simulink subsystem "ageing_model"  (R2022a)
settings: Solver=VariableStepAuto  StartTime=0.0  StopTime=10.0  RelTol=1e-3
undefined symbols (not defined in the file): Cn
settings Model: Creator=mateu  LastModifiedBy=mateu

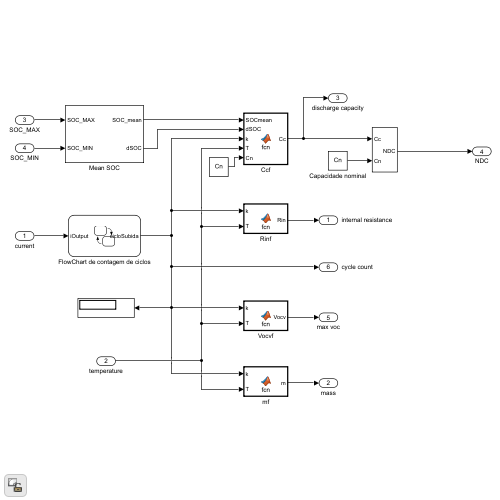
[thumbnail: Simulink's stored preview of the top-level diagram]
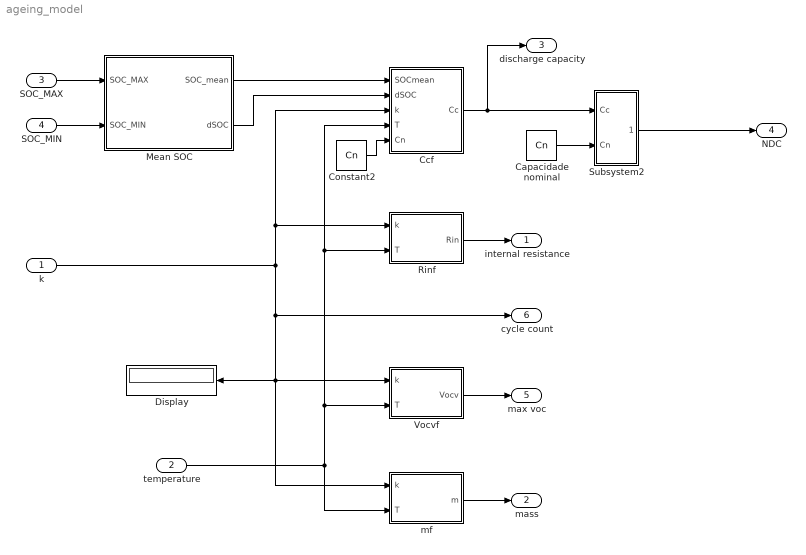
== system ageing_model ==
  k : Inport
  temperature : Inport  Port=2
  SOC_MAX : Inport  Port=3
  SOC_MIN : Inport  Port=4
  Capacidade nominal : Constant  Value=Cn
  Ccf : MATLAB Function  TreatAsAtomicUnit=on
  Constant2 : Constant  Value=Cn
  Display : Display
  Mean SOC : Subsystem
  Rinf : MATLAB Function  TreatAsAtomicUnit=on
  Subsystem2 : Subsystem
  Vocvf : MATLAB Function  TreatAsAtomicUnit=on
  mf : MATLAB Function  TreatAsAtomicUnit=on
  internal resistance : Outport
  mass : Outport  Port=2
  discharge capacity : Outport  Port=3
  NDC : Outport  Port=4
  max voc : Outport  Port=5
  cycle count : Outport  Port=6
  wires:
  Vocvf/1(Vocv) -> max voc/1
  temperature/1 -> Ccf/4(T), Rinf/2(T), Vocvf/2(T), mf/2(T)
  Rinf/1(Rin) -> internal resistance/1
  mf/1(m) -> mass/1
  Ccf/1(Cc) -> Subsystem2/1(Cc), discharge capacity/1
  Subsystem2/1(NDC) -> NDC/1
  Capacidade nominal/1 -> Subsystem2/2(Cn)
  Constant2/1 -> Ccf/5(Cn)
  SOC_MAX/1 -> Mean SOC/1(SOC_MAX)
  SOC_MIN/1 -> Mean SOC/2(SOC_MIN)
  Mean SOC/1(SOC_mean) -> Ccf/1(SOCmean)
  Mean SOC/2(dSOC) -> Ccf/2(dSOC)
  k/1 -> Vocvf/1(k), mf/1(k), Display/1, cycle count/1, Rinf/1(k), Ccf/3(k)

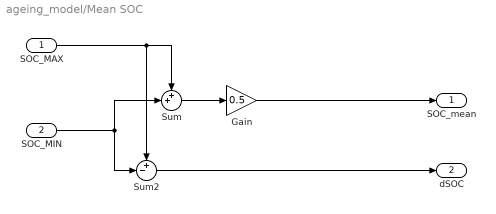
== system ageing_model/Mean SOC ==
  SOC_MAX : Inport
  SOC_MIN : Inport  Port=2
  Gain : Gain  Gain=0.5
  Sum : Sum  Inputs=++|
  Sum2 : Sum  Inputs=+-|
  SOC_mean : Outport
  dSOC : Outport  Port=2
  wires:
  Gain/1 -> SOC_mean/1
  Sum2/1 -> dSOC/1
  SOC_MAX/1 -> Sum2/1, Sum/1
  SOC_MIN/1 -> Sum2/2, Sum/2
  Sum/1 -> Gain/1

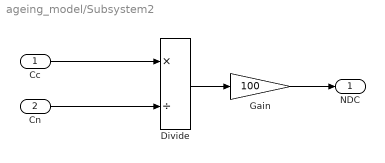
== system ageing_model/Subsystem2 ==
  Cc : Inport
  Cn : Inport  Port=2
  Divide : Product  Inputs=*/
  Gain : Gain  Gain=100
  NDC : Outport
  wires:
  Cc/1 -> Divide/1
  Gain/1 -> NDC/1
  Cn/1 -> Divide/2
  Divide/1 -> Gain/1

== matlab function ageing_model/Rinf ==
  data: k input; Rin output; T input
function Rin = fcn(k,T)

       x = (k-9000)/6326;
       y = (T-31.67)/10.57;
       
%        where x is normalized by mean 9000 and std 6326
%        and where y is normalized by mean 31.67 and std 10.57
% Coefficients (with 95% confidence bounds):
       p00 =    0.003956;%  (0.003728, 0.004184)
       p10 =   0.0006753;%  (0.0004339, 0.0009166)
       p01 =  -1.804e-05;%  (-0.0001419, 0.0001059)
       p20 =   0.0005921;%  (0.000144, 0.00104)
       p11 =   0.0002673;%  (4.651e-05, 0.0004881)
       p02 =   3.119e-05;%  (-0.0001491, 0.0002115)
       p30 =   0.0001137;%  (-7.891e-06, 0.0002354)
       p21 =   0.0002022;%  (0.0001025, 0.0003019)
       p12 =  -0.0002286;%  (-0.0003492, -0.0001081)
       p40 =  -1.788e-05;%  (-0.0002076, 0.0001718)
       p31 =  -1.552e-05;%  (-0.0001407, 0.0001096)
       p22 =  -0.0001674;%  (-0.0003125, -2.232e-05)

       %Linear model Poly42:
     Rin = p00 + p10*x + p01*y + p20*x^2 + p11*x*y + p02*y^2 + p30*x^3 + p21*x^2*y ...
                    + p12*x*y^2 + p40*x^4 + p31*x^3*y + p22*x^2*y^2;

       
% Goodness of fit:
%   SSE: 9.784e-08
%   R-square: 0.991
%   Adjusted R-square: 0.9746
%   RMSE: 0.0001277

== matlab function ageing_model/Ccf ==
  data: SOCmean input; dSOC input; k input; Cc output; T input; Cn input
function Cc = fcn(SOCmean, dSOC,k,T,Cn)
% Coeficients model Saxena2016
        k1 = 3.25;
        k2 = 3.25;
        k3 = -2.25;
% Coefficients (with 95% confidence bounds):
       p00 =       56.02;%  (53.93, 58.1)
       p10 =      -10.53;%  (-13.71, -7.36)
       p01 =       0.869;%  (-0.7052, 2.443)
       p20 =      -4.808;%  (-6.007, -3.609)
       p11 =      -1.445;%  (-2.534, -0.3554)
       p02 =      -1.223;%  (-2.763, 0.3179)
       p30 =      -2.931;%  (-4.53, -1.332)
       p21 =       -1.55;%  (-2.783, -0.3163)
       p12 =    -0.09181;%  (-1.677, 1.493)

       x = (k-9000)/6326;
       y = (T-31.67)/10.57;
       
%Linear model Poly32:
     fcn = p00 + p10*x + p01*y + p20*x^2 + p11*x*y + p02*y^2 + p30*x^3 + p21*x^2*y + p12*x*y^2;

     Cc = (100 - k1*SOCmean/100*(1+k2*dSOC/100+k3*(dSOC/100)^2) )/100*fcn
                    
%       where x is normalized by mean 9000 and std 6326
%       and where y is normalized by mean 31.67 and std 10.57


% Goodness of fit:
%   SSE: 29.68
%   R-square: 0.9934
%   Adjusted R-square: 0.9875
%   RMSE: 1.816

== matlab function ageing_model/Vocvf ==
  data: k input; Vocv output; T input
function Vocv = fcn(k,T)

%Coefficients (with 95% confidence bounds):
       p00 =       12.46;%  (12.4, 12.53)
       p10 =      0.2911;%  (0.2589, 0.3233)
       p01 =     0.03352;%  (-0.0006909, 0.06772)
       p20 =      0.0383;%  (-0.0004375, 0.07703)
       p11 =     0.02935;%  (-0.003774, 0.06248)
       p02 =    -0.01441;%  (-0.06418, 0.03537)

       x = (k-9000)/6326;
       y = (T-31.67)/10.57;
       
%Linear model Poly22:
     Vocv = p00 + p10*x + p01*y + p20*x^2 + p11*x*y + p02*y^2;
%       where x is normalized by mean 9000 and std 6326
%       and where y is normalized by mean 31.67 and std 10.57

%Goodness of fit:
%  SSE: 0.04454
%  R-square: 0.971
%  Adjusted R-square: 0.9588
%  RMSE: 0.06092

== matlab function ageing_model/mf ==
  data: k input; m output; T input
function m = fcn(k,T)

%Coefficients (with 95% confidence bounds):
       p00 =       19.64;%  (19.58, 19.69)
       p10 =     -0.5246;%  (-0.606, -0.4431)
       p01 =    -0.08727;%  (-0.1277, -0.04686)
       p20 =        0.06;%  (0.02923, 0.09077)
       p11 =    -0.04133;%  (-0.0693, -0.01337)
       p02 =    -0.04346;%  (-0.08301, -0.003916)
       p30 =     0.02928;%  (-0.01177, 0.07033)
       p21 =    -0.02198;%  (-0.05365, 0.009682)
       p12 =      0.0413;%  (0.0006076, 0.082)

       x = (k-9000)/6326;
       y = (T-31.67)/10.57;
       
% Linear model Poly32:
     m = p00 + p10*x + p01*y + p20*x^2 + p11*x*y + p02*y^2 + p30*x^3 + p21*x^2*y ...
                    + p12*x*y^2;
%        where x is normalized by mean 9000 and std 6326
%        and where y is normalized by mean 31.67 and std 10.57


% Goodness of fit:
%   SSE: 0.01956
%   R-square: 0.9946
%   Adjusted R-square: 0.9898
%   RMSE: 0.04662
